simulink model "progetto_tesi_def_AA"  (R2023b)
settings: Solver=ode1  StartTime=0.0  StopTime=inf  FixedStep=dt  RelTol=1e-3
values from neighbouring files (symbols this model uses):
  bias_acc = [0.1 , 0.1 , 0.1]    [model_params.m]
  degtoradianti = pi/180    (= 0.0174532925199)    [model_params.m]
  dt = 0.005    [model_params.m]
  gravity = -9.81007    [model_params.m]
  gyro_bias = gyro_bias_deg*degtoradianti    [model_params.m]
  noise_acc = 0.08 * gravity    (= -0.7848056)    [model_params.m]
  noise_gyro = 0.5* degtoradianti    (= 0.00872664625997)    [model_params.m]
  P_init = 1e-10 * eye(4)    [model_params.m]
  q_init = [1 0 0 0]'    [model_params.m]
undefined symbols (not defined in the file or in its folder): deg, m, s
libraries: simulink x3, qbmove_library x3, CP_library x1, dspstat3 x1, QB_pacer_lib x1
settings Model: Creator=ilari  LastModifiedBy=ilari

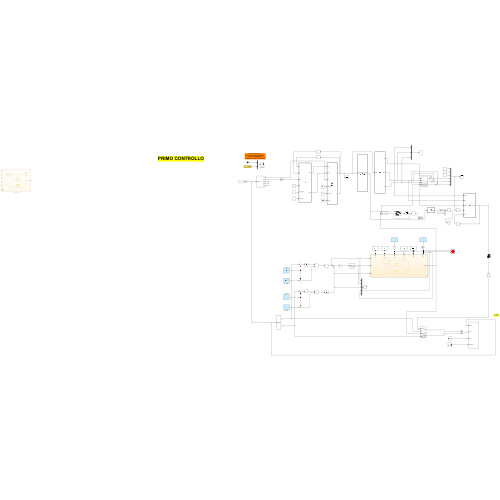
[thumbnail: Simulink's stored preview of the top-level diagram]
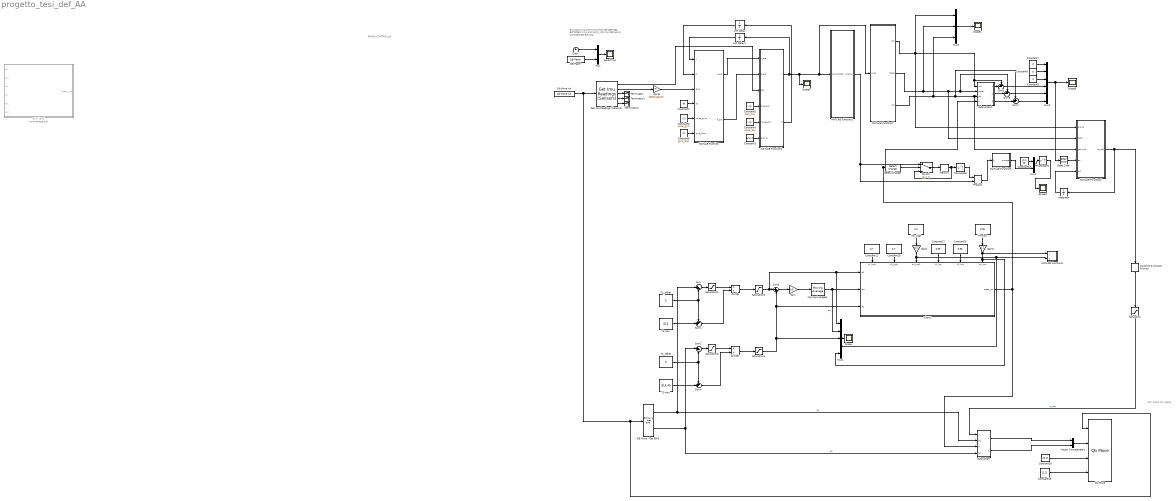
== system progetto_tesi_def_AA ==
  note: PRIMO CONTROLLO
  note: id 1: mano
      | id 2: polso
  note: Simulation sample time
      | MUST BE DEFINED BETWEEN
      | 1 ms and 0.6*N_IMU ms
      | PER EACH CONNECTED BOARD
  Chart1 : Stateflow chart  TreatAsAtomicUnit=on
      settings: PortSchema="{\"entries\":[{\"content\":{\"sides\":[{\"content\":{\"connectorIds\":[\"In1\",\"In2\",\"In3\"]},\"type\":\"ConnectorPlacement.EquallySpacedRectSide\",\"uuid\":\"4553bcbd-c641-47c7-8dbf-f79092e6ee81\"},{\"content\":{\"connectorIds\":[\"Out1\"],\"side\":\"RIGHT\"},\"type\":\"ConnectorPlacement.EquallySpacedRectSide\",\"uuid\":\"3da28b68-d93e-4f4c-9976-148e25354e99\"},{\"content\":{\"connectorIds\":[\"In8\",\"In6\",\"In4\",\"In9\",\"In7\",\"In5\"],\"side\":\"TOP\"},\"type\":\"ConnectorPlacement.EquallySpacedRectSide\",\"uuid\":\"8b0fc1d8-48d1-4cd9-90f0-88f64040c5cb\"}]},\"type\":\"ConnectorPlacement.EquallySpacedConnector\",\"uuid\":\"c86eeb24-54af-48fb-987a-3882c7f162b7\"}],\"packageUris\":[\"http://schema.mathworks.com/mf0/Connector/R2020b\"],\"version\":\"1.0\"}"
  Clock : Clock
  Constant1 : Constant  Value=dt
  Constant10 : Constant  Value=[0 0 0]'
  Constant11 : Constant  Value=0.7
  Constant15 : Constant  Value=0.7
  Constant17 : Constant  Value=0.55
  Constant18 : Constant  Value=[0 0]
  Constant19 : Constant  Value=[1 1]
  Constant2 : Constant  Value=noise_gyro
  Constant20 : Constant  Value=0.55
  Constant3 : Constant  Value=gravity
  Constant4 : Constant  Value=noise_acc
  Constant5 : Constant  Value=bias_acc
  Constant6 : Constant  Value=gyro_bias
  Constant7 : Constant  Value=0
  Constant8 : Constant  Value=0
  Constant9 : Constant  Value=0
  Coulomb & Viscous Friction : simulink/Discontinuities/Coulomb & Viscous Friction  offset=30  gain=1
  Dead Zone : DeadZone  LowerValue=-0.15  UpperValue=0.15
  Detect Change : simulink/Logic and Bit Operations/Detect Change  vinit=1  OutDataTypeStr=boolean
  Divide : Product  Inputs=*/
  Divide1 : Product  Inputs=*/
  Gain : Gain  Gain=0.5
  Gain1 : Gain  Gain=0.5
  Gain2 : Gain  Gain=1.2
  Gain6 : Gain  Gain=degtoradianti
  Get Imu Readings (Sensors) : CP_library/Get Imu Readings (Sensors)  ID=2  N_IMU=1  DAISY_CHAINING=off  ACC_UNITY=m/(s^2)  GYRO_UNITY=deg/s  MAG_UNITY=uT
      settings: SourceProductName=Centro Piaggio Library
  Integrator : Integrator
  MATLAB Function : MATLAB Function  TreatAsAtomicUnit=on
  MATLAB Function1 : MATLAB Function  TreatAsAtomicUnit=on
  MATLAB Function2 : MATLAB Function  TreatAsAtomicUnit=on
  MATLAB Function3 : MATLAB Function  TreatAsAtomicUnit=on
  MATLAB Function4 : MATLAB Function  TreatAsAtomicUnit=on
  MATLAB Function5 : MATLAB Function  TreatAsAtomicUnit=on
  MATLAB Function7 : MATLAB Function  TreatAsAtomicUnit=on
  Memory : Memory  InitialCondition=eye(3)
  Moving Average1 : dspstat3/Moving Average  Method=Sliding window  ForgettingFactorPort=off  SpecifyWindowLength=on  WindowLength=5  OverlapLength=4  AllowArbitraryInputLength=off  ForgettingFactor=0.9  SimulateUsing=Code generation
  Mux : Mux  Inputs=2
  Mux1 : Mux  Inputs=5
  Mux2 : Mux  Inputs=2
  Mux3 : Mux  Inputs=6
  Mux4 : Mux  Inputs=3
  Product : Product  Multiplication=Matrix(*)
  QB Move - Get EMG : qbmove_library/QB Move - Get EMG  ID=2  DAISY_CHAINING=off
      settings: SourceProductName=Qb Move Library
  QB Pacer : QB_pacer_lib/QB Pacer  simTimePerRealTime=1
      settings: SourceProductName=QB Pacer
  Qb Move : qbmove_library/Qb Move  ID=[1 2]  ACTIVE_COMM_DIRECTIONS=Tx  CONTROL_MODE=Prime Movers Positions  DAISY_CHAINING=off  MAX_ANG=0  SW_LIMIT=inf  OFFSET=0  ACTIVATE=off  WDT=0.0  UNIT=TICK
      settings: LibrarySourceBlock=qbmove_library/qbmove  SourceProductName=Qb Move Library
  Qb Move Init : qbmove_library/Qb Move Init  NUMBER_OF_COM='COM9'  BAUD_RATE_COM=2000000
      settings: SourceProductName=Qb Move Library
  Saturation : Saturate  UpperLimit=100  LowerLimit=-100
  Saturation1 : Saturate  UpperLimit=1024  LowerLimit=0
  Saturation2 : Saturate  UpperLimit=1  LowerLimit=0
  Saturation3 : Saturate  UpperLimit=1024  LowerLimit=0
  Saturation4 : Saturate  UpperLimit=1  LowerLimit=0
  Scope{,1..2,4..5} (5 alike) : Scope
  Subsystem : Subsystem
  Subsystem1 : Subsystem
  Sum : Sum  Inputs=|+-
  Sum1 : Sum  Inputs=-+|
  Sum2 : Sum  Inputs=|+-
  Sum3 : Sum  Inputs=+-|
  Sum4 : Sum  Inputs=-+|
  Sum5 : Sum  Inputs=|++
  Sum6 : Sum  Inputs=+-|
  Sum7 : Sum  Inputs=+-|
  Switch : Switch  Criteria=u2 > Threshold  SaturateOnIntegerOverflow=off  InputSameDT=off
  T1 max : Constant  Value=613
  T1_offset : Constant  Value=2
  T2 max : Constant  Value=815.45
  T2_offset : Constant  Value=2
  Terminator : Terminator
  Terminator1 : Terminator
  Terminator2 : Terminator
  Tm_high : Constant  Value=0.2
  Tm_low : Constant  Value=0.05
  Transpose1 : Math  Operator=transpose
  Transpose2 : Math  Operator=transpose
  Unit Delay : UnitDelay  InitialCondition=P_init  SampleTime=-1  HasFrameUpgradeWarning=on
  Unit Delay1 : UnitDelay  InitialCondition=q_init  SampleTime=-1  HasFrameUpgradeWarning=on
  Vector Concatenate1 : Concatenate
  only I level : Stateflow chart  Commented=on  TreatAsAtomicUnit=on
  pacerTime : Scope
  wires:
  Clock/1 -> Mux/1
  Mux/1 -> pacerTime/1
  QB Pacer/1 -> Mux/2
  Get Imu Readings (Sensors)/5 -> Terminator2/1
  Get Imu Readings (Sensors)/4 -> Terminator1/1
  Get Imu Readings (Sensors)/3 -> Terminator/1
  Get Imu Readings (Sensors)/2 -> Gain6/1
  MATLAB Function/1(x_pre) -> MATLAB Function1/1(x_pre)
  MATLAB Function/2(P_pre) -> MATLAB Function1/2(P_pre)
  Get Imu Readings (Sensors)/1 -> MATLAB Function1/3(acc)
  MATLAB Function1/1(x) -> Scope2/1, MATLAB Function2/1(quat), MATLAB Function7/1(quat), Unit Delay1/1
  Unit Delay1/1 -> MATLAB Function/1(x)
  MATLAB Function1/2(P) -> Unit Delay/1
  Unit Delay/1 -> MATLAB Function/2(P)
  Gain6/1 -> MATLAB Function/3(gyro)
  Constant1/1 -> MATLAB Function/4(dt)
  Constant2/1 -> MATLAB Function/5(noise_gyro)
  Constant3/1 -> MATLAB Function1/6(gravity)
  Constant4/1 -> MATLAB Function1/5(noise_acc)
  Constant5/1 -> MATLAB Function1/4(bias_acc)
  Constant6/1 -> MATLAB Function/6(gyro_bias)
  Integrator/1 -> MATLAB Function4/5(qrx)
  QB Move - Get EMG/2 -> Subsystem/4(e2), Sum2/1  "e2"
  QB Move - Get EMG/1 -> Subsystem/2(e1), Sum/1  "e1"
  MATLAB Function4/1(qr_dot) -> Integrator/1, Coulomb & Viscous Friction/1
  Constant18/1 -> Qb Move/3
  Constant19/1 -> Qb Move/4
  Qb Move Init/1 -> Get Imu Readings (Sensors)/1, QB Move - Get EMG/1, Qb Move/1
  Vector Concatenate1/1 -> Qb Move/2
  Switch/1 -> Memory/1
  Memory/1 -> Transpose2/1, Switch/3
  Product/1 -> MATLAB Function5/1(R)
  Constant10/1 -> Mux2/1
  Mux2/1 -> Transpose1/1
  Transpose1/1 -> Scope4/1
  MATLAB Function7/3(psi) -> MATLAB Function4/3(gamma), Subsystem1/3(psi), Sum7/1, Mux4/3
  MATLAB Function7/2(theta) -> MATLAB Function4/2(beta), Subsystem1/2(theta), Sum6/1, Mux4/2
  MATLAB Function7/1(phi) -> Sum3/1, Subsystem1/1(phi), Mux4/1, MATLAB Function4/1(alpha)
  Sum/1 -> Saturation1/1
  Saturation1/1 -> Divide/1
  T1_offset/1 -> Sum1/1, Sum/2
  T1 max/1 -> Sum1/2
  Sum1/1 -> Divide/2
  Divide/1 -> Saturation2/1
  T2_offset/1 -> Sum4/1, Sum2/2
  Sum2/1 -> Saturation3/1
  Saturation3/1 -> Divide1/1
  Divide1/1 -> Saturation4/1
  Sum4/1 -> Divide1/2
  T2 max/1 -> Sum4/2
  Saturation2/1 -> Mux1/1, Chart1/1(e1), Sum5/1
  Saturation4/1 -> Mux1/3, Chart1/3(e2), Sum5/2
  Sum5/1 -> Gain/1
  Gain/1 -> Moving Average1/1
  Moving Average1/1 -> Mux1/2, Chart1/2(em)  "em"
  Saturation/1 -> Subsystem/1(qr_dot)  "qr_dot"
  Mux1/1 -> Scope/1
  Constant11/1 -> Chart1/8(t1_high)
  Constant20/1 -> Chart1/7(t2_low)
  Constant17/1 -> Chart1/9(t1_low)
  Tm_high/1 -> Gain1/1
  Constant15/1 -> Chart1/6(t2_high)
  Tm_low/1 -> Gain2/1
  Coulomb & Viscous Friction/1 -> Saturation/1
  Constant9/1 -> Mux3/3
  Sum6/1 -> Mux3/5
  Subsystem1/2(Output1) -> Sum6/2
  Sum7/1 -> Mux3/6
  Constant8/1 -> Mux3/2
  Subsystem1/1(Output) -> Sum3/2
  Constant7/1 -> Mux3/1
  Sum3/1 -> Mux3/4
  Subsystem1/3(Output2) -> Sum7/2
  Mux3/1 -> Dead Zone/1, Scope5/1
  Subsystem/1(Hand) -> Vector Concatenate1/1
  Subsystem/2(Wrist) -> Vector Concatenate1/2
  Gain1/1 -> MATLAB Function3/2(Tm_high), Mux1/4, Chart1/4(tm_high)
  Gain2/1 -> Mux1/5, Chart1/5(tm_low), MATLAB Function3/1(Tm_low)
  MATLAB Function5/1(omega) -> Mux2/2
  Mux4/1 -> Scope1/1
  Chart1/1(state_var) -> Subsystem/3(state_var), Subsystem1/4(reset pose), Detect Change/1
  Detect Change/1 -> Switch/2
  MATLAB Function2/1(Rotation_matrix) -> Product/2, Switch/1
  Transpose2/1 -> Product/1
  Dead Zone/1 -> MATLAB Function4/4(ec)

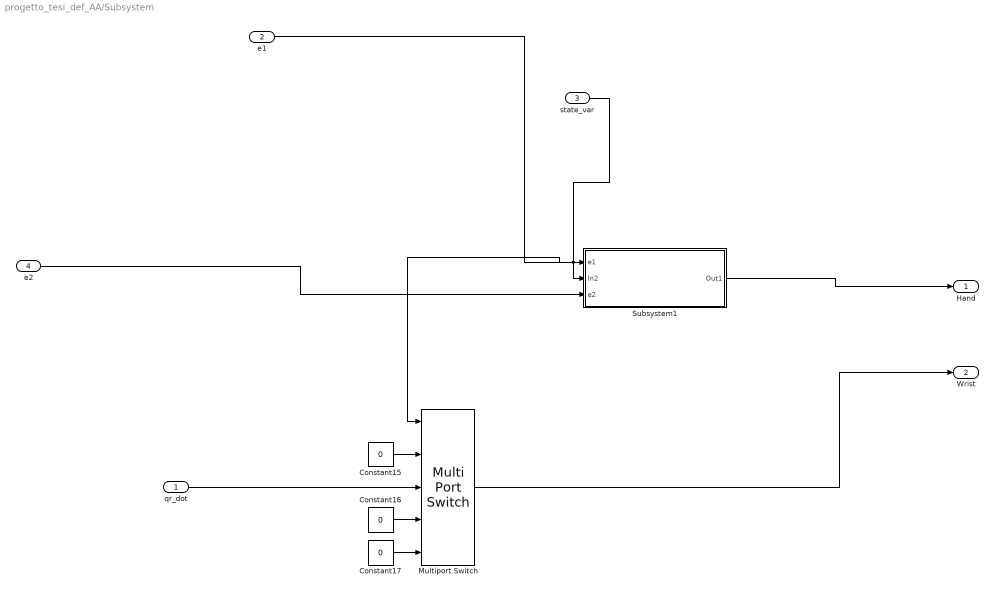
== system progetto_tesi_def_AA/Subsystem ==
  qr_dot : Inport
  e1 : Inport  Port=2
  state_var : Inport  Port=3
  e2 : Inport  Port=4
  Constant15 : Constant  Value=0
  Constant16 : Constant  Value=0
  Constant17 : Constant  Value=0
  Multiport Switch : MultiPortSwitch  DataPortOrder=Zero-based contiguous  Inputs=4  zeroidx=on  SaturateOnIntegerOverflow=off  InputSameDT=off
  Subsystem1 : Subsystem
  Hand : Outport
  Wrist : Outport  Port=2
  wires:
  state_var/1 -> Multiport Switch/1, Subsystem1/2(In2)
  Multiport Switch/1 -> Wrist/1
  Constant17/1 -> Multiport Switch/5
  Subsystem1/1(Out1) -> Hand/1
  Constant16/1 -> Multiport Switch/4
  Constant15/1 -> Multiport Switch/2
  e2/1 -> Subsystem1/3(e2)
  e1/1 -> Subsystem1/1(e1)
  qr_dot/1 -> Multiport Switch/3

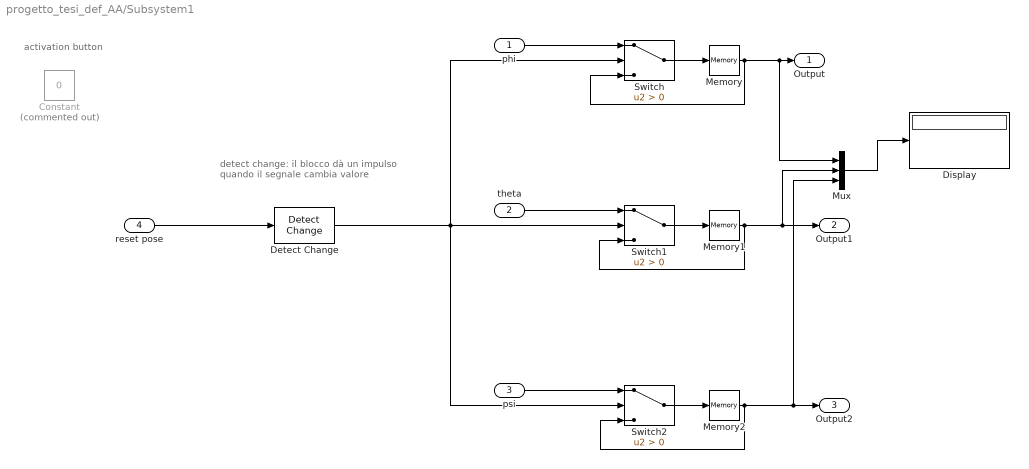
== system progetto_tesi_def_AA/Subsystem1 ==
  note: detect change: il blocco dà un impulso
      |  quando il segnale cambia valore
  note: activation button
  phi : Inport
  theta : Inport  Port=2
  psi : Inport  Port=3
  reset pose : Inport  Port=4
  Constant : Constant  Commented=on  Value=0
  Detect Change : simulink/Logic and Bit Operations/Detect Change  vinit=0  OutDataTypeStr=boolean
  Display : Display
  Memory : Memory
  Memory1 : Memory
  Memory2 : Memory
  Mux : Mux  Inputs=3
  Switch : Switch  Criteria=u2 > Threshold  SaturateOnIntegerOverflow=off  InputSameDT=off
  Switch1 : Switch  Criteria=u2 > Threshold  SaturateOnIntegerOverflow=off  InputSameDT=off
  Switch2 : Switch  Criteria=u2 > Threshold  SaturateOnIntegerOverflow=off  InputSameDT=off
  Output : Outport
  Output1 : Outport  Port=2
  Output2 : Outport  Port=3
  wires:
  Memory/1 -> Switch/3, Mux/1, Output/1
  Switch1/1 -> Memory1/1
  Memory1/1 -> Switch1/3, Output1/1, Mux/2
  Switch2/1 -> Memory2/1
  Memory2/1 -> Switch2/3, Output2/1, Mux/3
  Switch/1 -> Memory/1
  phi/1 -> Switch/1
  theta/1 -> Switch1/1
  psi/1 -> Switch2/1
  Detect Change/1 -> Switch/2, Switch2/2, Switch1/2
  reset pose/1 -> Detect Change/1
  Mux/1 -> Display/1

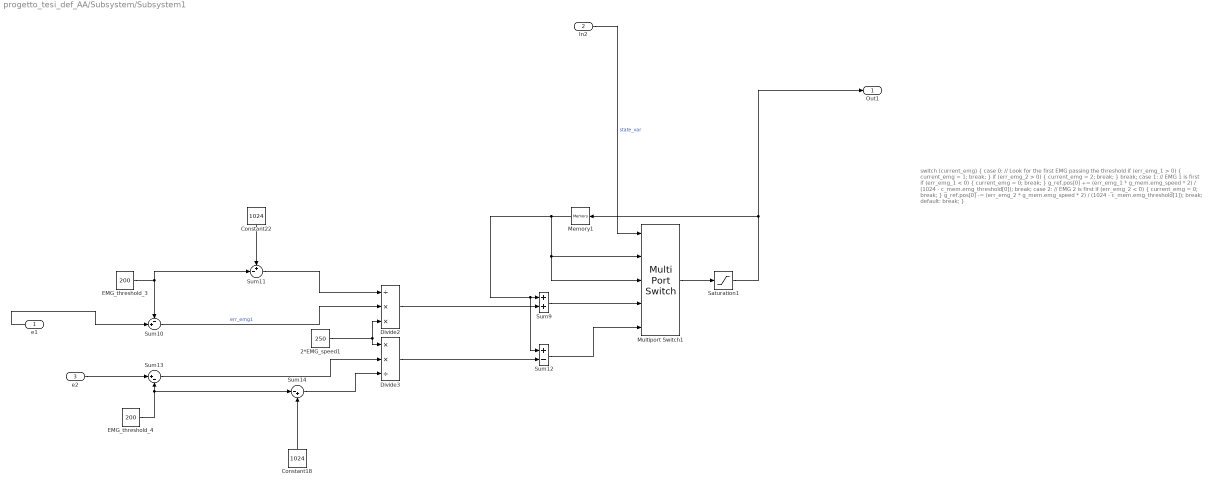
== system progetto_tesi_def_AA/Subsystem/Subsystem1 ==
  note: switch (current_emg) {
      | case 0:
      | // Look for the first EMG passing the threshold
      | if (err_emg_1 > 0) {
      | current_emg = 1;
      | break;
      | }
      | if (err_emg_2 > 0) {
      | current_emg = 2;
      | break;
      | }
      | break;
      |
      | case 1:
      | // EMG 1 is first
      | if (err_emg_1 < 0) {
      | current_emg = 0;
      | break;
      | }
      | g_ref.pos[0] += (err_emg_1 * g_mem.emg_speed * 2) / (1024 - c_mem.emg_threshold[0]);
      | break;
      |
      | case 2:
      | // EMG 2 is first
      | if (err_emg_2 < 0) {
      | current_emg = 0;
      | break;
      | }
      | g_ref.pos[0] -= (err_emg_2 * g_mem.emg_speed * 2) / (1024 - c_mem.emg_threshold[1]);
      | break;
      |
      | default:
      | break;
      | }
  e1 : Inport
  In2 : Inport  Port=2
  e2 : Inport  Port=3
  2*EMG_speed1 : Constant  Value=250
  Constant18 : Constant  Value=1024
  Constant22 : Constant  Value=1024
  Divide2 : Product  Inputs=/**
  Divide3 : Product  Inputs=**/
  EMG_threshold_3 : Constant  Value=200
  EMG_threshold_4 : Constant  Value=200
  Memory1 : Memory
  Multiport Switch1 : MultiPortSwitch  DataPortOrder=Zero-based contiguous  Inputs=4  zeroidx=on  SaturateOnIntegerOverflow=off  InputSameDT=off
  Saturation1 : Saturate  UpperLimit=17500  LowerLimit=0
  Sum10 : Sum  Inputs=-+|
  Sum11 : Sum  Inputs=+-|
  Sum12 : Sum  Inputs=+-
  Sum13 : Sum  Inputs=|+-
  Sum14 : Sum  Inputs=|-+
  Sum9 : Sum
  Out1 : Outport
  wires:
  Multiport Switch1/1 -> Saturation1/1
  Memory1/1 -> Multiport Switch1/2, Multiport Switch1/3, Sum12/1, Sum9/1
  e1/1 -> Sum10/2
  Sum11/1 -> Divide2/1
  Sum9/1 -> Multiport Switch1/4
  Saturation1/1 -> Out1/1, Memory1/1
  Divide2/1 -> Sum9/2
  Divide3/1 -> Sum12/2
  Sum14/1 -> Divide3/3
  EMG_threshold_3/1 -> Sum11/2, Sum10/1
  EMG_threshold_4/1 -> Sum14/1, Sum13/2
  Constant18/1 -> Sum14/2
  2*EMG_speed1/1 -> Divide3/1, Divide2/3
  Sum13/1 -> Divide3/2
  e2/1 -> Sum13/1
  Sum12/1 -> Multiport Switch1/5
  Sum10/1 -> Divide2/2  "err_emg1"
  Constant22/1 -> Sum11/1
  In2/1 -> Multiport Switch1/1  "state_var"

== matlab function progetto_tesi_def_AA/MATLAB Function4 ==
  data: alpha input; beta input; gamma input; qr_dot output; ec input size=[1 6]; qrx input
% function qr_dot = wrist_control(ec, Jre , Jhc , Jhe , kc)
% ec = ec'; %deve essere 6x1
% Jre_i = pinv(Jre);
% Jhe_i = pinv(Jhe);
% qr_dot = -Jre_i*(pinv(Jhc*Jhe_i))*kc*ec ;
% 
% end

function qr_dot = wrist_control(alpha, beta, gamma, ec, qrx )

ec = ec';
% alpha = ec(4); %phi
% beta = ec(5);  %theta
% gamma = ec(6); %psi
kc = 100 ;
l1=0.3; %[m]
lw = 0.1; %[m]
Rxyz =[cos(beta)*cos(gamma) , (sin(alpha)*sin(beta)*cos(gamma))-(cos(alpha)*sin(gamma)), (cos(alpha)*sin(beta)*cos(gamma))+(sin(alpha)*sin(gamma));
       cos(beta)*sin(gamma) , (sin(alpha)*sin(beta)*sin(gamma))+(cos(alpha)*cos(gamma)), (cos(alpha)*sin(beta)*sin(gamma))-(sin(alpha)*cos(gamma));
       -sin(beta)           , sin(alpha)*cos(beta)                                     ,  cos(alpha)*cos(beta)                                     ];  

Rx_qrx = [1 0 0; 0 cos(qrx) -sin(qrx); 0 sin(qrx) cos(qrx)];

Rxyzx = Rxyz*Rx_qrx;

vector_p = [-l1 0 0]';
vector_p_tras = Rxyz*vector_p + Rxyzx*[-lw ; 0 ; 0];
z1 = Rxyzx(:,1);
z2 = Rxyzx(:,2);
z3 = Rxyzx(:,3);

Jrc = [0 0 0 0 0 0]';
Jhc = [zeros(3,3); Rxyz];
Jre = [0;0;0;z1];
Jhe = [cross(z1,vector_p_tras) , cross(z2,vector_p_tras) , cross(z1,vector_p_tras); z1, z2, z3];

Jre_i = pinv(Jre);
Jhe_i = pinv(Jhe);
% K=-Jre_i*(pinv(Jhc*Jhe_i))*kc;

qr_dot = -Jre_i*(pinv(Jhc*Jhe_i))*kc*ec;

== matlab function progetto_tesi_def_AA/MATLAB Function3 ==
  data: Tm_low input; Tm_high input
function check_errors(Tm_low,Tm_high)

if Tm_low >Tm_high
    error('The provided thresholds cannot represent a real situation');
end
end

== stateflow chart progetto_tesi_def_AA/only I level ==
  note: rest
  note: polso on
  state state0
    entry: state_var = 0;
  state state1
    entry: state_var=1;
  note: mano chiusa
  state state2
    entry: state_var=2;
  note: mano aperta
  state state3
    entry: state_var=3;
  (default) -> state0
  state0 -> state1 [order 1] : [em>tm && e1<th1 && e2<th2 && after(2, sec)]
  state1 -> state0 : [em<tm && after(2, sec)]
  state3 -> state0 : [em<tm && e2<th2 && after(2, sec)]
  state0 -> state3 [order 3] : [em>tm && e2>th2 && after(2, sec)]
  state0 -> state2 [order 2] : [em>tm && e1>th1 && after(2, sec)]
  state2 -> state0 : [em<tm && e1<th1 && after(2, sec)]
  data: e1 input; em input size=1; e2 input; tm input; th1 input; state_var output; th2 input

== matlab function progetto_tesi_def_AA/MATLAB Function5 ==
  data: R input; omega output
function omega  = fcn(R)

aa = rotm2axang(R);
omega = aa(1:3)'*aa(4);

end

== matlab function progetto_tesi_def_AA/MATLAB Function7 ==
  data: quat input; phi output; theta output; psi output
function [phi, theta , psi] = quaternions2euler(quat)

q0 = quat(1);
q1 = quat(2);
q2 = quat(3);
q3 = quat(4);

phi = atan2(2*(q2*q3 + q0*q1), q0^2 -q1^2 -q2^2 +q3^2);
theta = -asin(2*(q1*q3 -q0*q2));
psi = atan2(2*(q1*q2 + q0*q3), q0^2 + q1^2 -q2^2 -q3^2);

end

== matlab function progetto_tesi_def_AA/MATLAB Function1 ==
  data: x_pre input; x output size=[4 1]; P_pre input; acc input; bias_acc input size=[1 3]; noise_acc input; gravity input; P output
function [x , P] = EKF_update(x_pre , P_pre , acc  , bias_acc , noise_acc,  gravity)

% Inizializzazione variabili di output
x = x_pre;
P = P_pre;

%correzione delle letture
acc = acc - bias_acc;
%mag = mag - bias_mag;

%Update accelerometro
if norm(acc) ~= 0
    acc_norm = acc'/norm(acc);
else
    acc_norm = acc'; %[3x1]
end

%utilizzo formula gravità come modello di osservazione

acc_prediction = [ 2*(x_pre(2)*x_pre(4)-x_pre(1)*x_pre(3));
                   2*(x_pre(3)*x_pre(4)+x_pre(1)*x_pre(2));
                   x_pre(1)^2-x_pre(2)^2-x_pre(3)^2+x_pre(4)^2]; %[3x1]

%calcolo del residuo (innovazione)
y_acc = acc_norm - acc_prediction;  %[3x1]

% derivo modello di osservazione per ottenere la matrice H
H_acc =   2 * [-x_pre(3)    x_pre(4)    -x_pre(1)   x_pre(2); 
            x_pre(2)    x_pre(1)     x_pre(4)   x_pre(3); 
            x_pre(1)   -x_pre(2)    -x_pre(3)   x_pre(4)]; %[3x4]

% Rumore di misura R
if norm(acc) ~= 0 
    R_acc_internal = (noise_acc / norm(acc))^2 * eye(3);
    R_acc_external = (1-gravity/norm(acc))^2 * eye(3);
    R_acc = R_acc_internal + R_acc_external;
else 
    R_acc = eye(3);
end

%  fase di Update accelerometro

S_acc = H_acc * P_pre * H_acc' + R_acc; %[3x3]
K_acc = P_pre * H_acc' / S_acc; %[4x3]
x = x_pre + K_acc * y_acc; %[4x1]
P = (eye(4) - K_acc * H_acc) * P_pre; %[4x4]

% %% Update magnetometro
% 
% if norm(mag) ~= 0
%     mag_norm = mag'/norm(mag);
% else
%     mag_norm = mag'; %[3x1]
% end
% 
% mag_prediction = [ 2*(x_pre(2)*x_pre(4)+x_pre(1)*x_pre(3));
%                    2*(x_pre(3)*x_pre(4)-x_pre(1)*x_pre(2));
%                    x_pre(1)^2-x_pre(2)^2-x_pre(3)^2+x_pre(4)^2]; %[3x1]
% 
% y_mag = mag_norm - mag_prediction;  %[3x1]
% 
% H_mag = 2 * [ x_pre(3)    x_pre(4)     x_pre(1)    x_pre(2);
%              -x_pre(2)    x_pre(1)    -x_pre(4)    x_pre(3);
%               x_pre(1)   -x_pre(2)    -x_pre(3)    x_pre(4)]; %[3x4]
% 
% R_mag = eye(3);
% 
% if norm(mag) ~= 0
%     R_mag = (noise_mag / norm(mag))^2 * eye(3);
% end
% 
% S_mag = H_mag * P * H_mag' + R_mag; %[3x3]
% K_mag = P * H_mag' / S_mag; %[4x3]
% x = x + K_mag * y_mag; %[4x1]
% P = (eye(4) - K_mag * H_mag) * P;


if norm(x) ~= 0
    x = x/norm(x);
else


end

== matlab function progetto_tesi_def_AA/MATLAB Function ==
  data: x input size=[4 1]; x_pre output; P input; gyro input; P_pre output; dt input; noise_gyro input; gyro_bias input
function [x_pre, P_pre] = EKF_prediction(x, P, gyro, dt, noise_gyro, gyro_bias)

    % x: stato corrente [ q0 q1 q2 q3 bx by bz] [7x1]
    %pre = predetto

    % P: matrice covarianza dello stato

    % z: misurazione (accelerometro e magnetometro)

    % gyro (u) ingresso di controllo (dati del giroscopio) [wx wy wz] [p q r]

    % Q: covarianza del rumore di processo

    % R: covarianza del rumore di misura

   

   %% STATO
       
    %       |   q0    |
    %       |   q1    |
    %  x =  |   q2    |
    %       |   q3    |

    %% Predizione

   %   x(k+1) ~= x(k) + f(x(k),0)*dt
   % 
   % q0 = state_hat(1);
   % q1 = state_hat(2);
   % q2 = state_hat(3);
   % q3 = state_hat(4);

   % correggo le misure di giroscopio 

   wx = gyro(1) - gyro_bias(1);
   wy = gyro(2) - gyro_bias(2);
   wz = gyro(3) - gyro_bias(3);

   % wx = gyro(1);
   % wy = gyro(2);
   % wz = gyro(3);


   
   Omega =[ 0   -wx  -wy  -wz;
            wx   0    wz   -wy; 
            wy  -wz   0     wx;
            wz   wy  -wx    0  ];


   F = eye(4) + dt * 0.5 * Omega ;



   % dot_matrix = [0     -(wx-bx)     -(wy-by)    -(wz-bz)   0 0 0;
   %              (wx-bx)     0        (wz-bz)    -(wy-by)   0 0 0;
   %              (wy-by) -(wz-bz)        0        (wx-bz)   0 0 0;
   %              (wz-bz)  (wy-by)     -(wx-bx)       0      0 0 0;
   %                0         0            0          0      0 0 0;
   %                0         0            0          0      0 0 0;
   %                0         0            0          0      0 0 0]; %[7x7]

  
  % state_hat_pre = state_hat + 0.5*dt*dot_matrix*state_hat  %stato predetto
  
  
  % Compute the process noise Q %capire da dove viene la formula

    G = [-x(2)  -x(3)  -x(4); 
          x(1)  -x(4)   x(3); 
          x(4)   x(1)  -x(2); 
         -x(3)   x(2)   x(1)] / 2;

    Q = (noise_gyro * dt)^2 * (G * G');
    
    % Propagate the state and covariance
    x_pre = F * x;
    x_pre = x_pre / norm(x_pre);    % Normalize the quaternion
    P_pre = F * P * F' + Q;
    

end

== matlab function progetto_tesi_def_AA/MATLAB Function2 ==
  data: quat input; Rotation_matrix output
function Rotation_matrix = Quat2rot(quat)

% x = quat(1);
% y = quat(2);
% w = quat(3);
% z = quat(4);
% Rotating_matrix = [(1 - 2*(y^2 + z^2)) , 2*(x*y - w*z) , 2*(w*y + x*z);
%                     2*(x*y + w*z) , (1 - 2*(x^2 + z^2)) , 2*(y*z - w*x);
%                     2*(x*z - w*y) , 2*(w*x + y*z) , (1 - 2*(x^2 + y^2))];

Rotation_matrix = quat2rotm(quat');

end

== stateflow chart progetto_tesi_def_AA/Chart1 ==
  state state0
    entry: state_var = 0;
    t_high =0;
    during:
    if (em > tm_high)
    t_high = t_high + dt;
    else
    t_high = 0;
    end
  note: rest
  note: polso on
  state state1
    entry: state_var=1;
  note: mano chiusa
  state state2
    entry: state_var=2;
  note: mano aperta
  state state3
    entry: state_var=3;
  (default) -> state0
  state0 -> state1 [order 1] : [t_high>0.3]
  state1 -> state0 [order 1] : [em<tm_low & after(1 ,sec)]
  state1 -> state3 [order 2] : [e2>t2_high && after(1, sec)]
  state3 -> state1 [commented out] : [em>tm & e2<t2_low]
  state2 -> state1 [commented out] : [em>tm &e1<t1_low]
  state1 -> state2 [order 3] : [e1>t1_high & after(1, sec)]
  state3 -> state0 : [ e2<t2_low]
  state0 -> state3 [order 3] : [ e2>t2_high]
  state0 -> state2 [order 2] : [e1>t1_high]
  state2 -> state0 : [ e1<t1_low]
  data: e1 input; em input size=1; e2 input; state_var output; tm_high input; tm_low input; t2_high input; t2_low input; t1_high input; t1_low input; dt parameter; t_high local
